simulink model "CUD_10m"  (R2019a)
settings: Solver=VariableStepAuto  StartTime=1.0  StopTime=144  RelTol=1e-3
values from neighbouring files (symbols this model uses):
  altezza = [0,0,0,0,0,0,0,0,0,0,0,0,0,0,0,0,0,0,0,0,0,0,0,0,0,0,0,0,0,0,0,0,0,0,0,0,0,0,0.81,2.62,4.43,6.26,8.1,9.94,11.79,13.65,15.51,17.37,19.23,21.1,22.95,24.81,26.66,28.49,30.32,32.14,33.94,35.73,37.49,39.23,40.94,42.62,44.27,45.87,47.43,48.94,50.39,51.77,53.08,54.3,55.44,56.47,57.39,58.18,58.85,59.37,59.74,59.96,60.02,59.93,59.67,59.27,58.71,58.02,57.2,56.25,55.2,54.05,52.8,51.48,50.08,48.62,47.1,45.53, ...(+192 chars)    [controllo_utenze_domestiche.m]
  area = pi*l_pale^2/4    (= 78.5398163397)    [controllo_utenze_domestiche.m]
  asciugacapelli = utenze(7,:)    [controllo_utenze_domestiche.m]
  azimut = [0,0,0,0,0,0,0,0,0,0,0,0,0,0,0,0,0,0,0,0,0,0,0,0,0,0,0,0,0,0,0,0,0,0,0,0,0,0,74.76,76.41,78.06,79.69,81.32,82.95,84.58,86.21,87.86,89.51,91.18,92.88,94.59,96.34,98.12,99.94,101.81,103.73,105.7,107.74,109.85,112.05,114.33,116.72,119.21,121.83,124.58,127.47,130.51,133.73,137.12,140.7,144.46,148.43,152.58,156.92,161.43,166.09,170.86,175.71,180.61,185.49,190.33,195.08,199.71,204.18,208.48,212.59,216.5 ...(+274 chars)    [controllo_utenze_domestiche.m]
  computer = utenze(9,:)    [controllo_utenze_domestiche.m]
  condizionatori = utenze(4,:)    [controllo_utenze_domestiche.m]
  console = utenze(13,:)    [controllo_utenze_domestiche.m]
  Cp = 0.22    [controllo_utenze_domestiche.m]
  densita = 1.225    [controllo_utenze_domestiche.m]
  fornitura = 3000    [controllo_utenze_domestiche.m]
  forno = utenze(2,:)    [controllo_utenze_domestiche.m]
  frigorifero = utenze(3,:)    [controllo_utenze_domestiche.m]
  irraggiamento = [0,0,0,0,0,0,0,0,0,0,0,0,0,0,0,0,0,0,0,0,0,0,0,0,0,0,0,0,0,0,0,0,0,0,0,0,0,0,0,0,0,0,0,1000,1000,1000,1000,1000,1000,1000,1000,1000,1000,1000,1000,1000,1000,1000,1000,1000,1000,1000,1000,1000,1000,1000,1000,1000,1000,1000,1000,1000,1000,1000,1000,1000,1000,1000,1000,1000,1000,1000,1000,1000,1000,1000,1000,1000,1000,1000,1000,1000,1000,1000,1000,1000,1000,1000,1000,1000,1000,1000,1000,1000,1000,100 ...(+102 chars)    [controllo_utenze_domestiche.m]
  lavastoviglie = utenze(6,:)    [controllo_utenze_domestiche.m]
  lavatrice = utenze(1,:)    [controllo_utenze_domestiche.m]
  luci = utenze(12,:)    [controllo_utenze_domestiche.m]
  microonde = utenze(10,:)    [controllo_utenze_domestiche.m]
  N_cell = 5    [controllo_utenze_domestiche.m]
  N_comp = 3    [controllo_utenze_domestiche.m]
  N_luci = 8    [controllo_utenze_domestiche.m]
  N_pale = 4    [controllo_utenze_domestiche.m]
  N_pann = 10    [controllo_utenze_domestiche.m]
  N_tel = 3    [controllo_utenze_domestiche.m]
  pot_asciu = 2000    [controllo_utenze_domestiche.m]
  pot_comp = 150    [controllo_utenze_domestiche.m]
  pot_cond = 50    [controllo_utenze_domestiche.m]
  pot_cons = 250    [controllo_utenze_domestiche.m]
  pot_forno = 1500    [controllo_utenze_domestiche.m]
  pot_frigo = 25    [controllo_utenze_domestiche.m]
  pot_lav = 2100    [controllo_utenze_domestiche.m]
  pot_lavast = 670    [controllo_utenze_domestiche.m]
  pot_luci = 5    [controllo_utenze_domestiche.m]
  pot_micro = 800    [controllo_utenze_domestiche.m]
  pot_ric = 3    [controllo_utenze_domestiche.m]
  pot_scald = 1500    [controllo_utenze_domestiche.m]
  pot_ste = 150    [controllo_utenze_domestiche.m]
  pot_tel = 55    [controllo_utenze_domestiche.m]
  rend_sol = 0.2    [controllo_utenze_domestiche.m]
  ricariche_cell = utenze(14,:)    [controllo_utenze_domestiche.m]
  scaldabagno = utenze(11,:)    [controllo_utenze_domestiche.m]
  sfasamento = -180    [controllo_utenze_domestiche.m]
  stereo_dvd = utenze(8,:)    [controllo_utenze_domestiche.m]
  sup_pann = 1.5    [controllo_utenze_domestiche.m]
  televisore = utenze(5,:)    [controllo_utenze_domestiche.m]
  vel_vento = [1.3, 1.4, 1.5, 1.7, 1.2, 2.0, 2.1, 1.8, 1.7, 1.5, 1.9, 2.0, 2.2, 2.1, 1.9, 1.7, 1.9, 2.1, 2.2, 2.0, 2.3, 2.1, 2.0, 1.9, 2.1, 2.4, 2.2, 2.2, 2.1, 1.9, 1.5, 1.3, 1.1, 0.9, 1.0, 0.7, 0.8, 0.9, 0.6, 0.9, 1.0, 1.1, 1.2, 1.3, 1.4, 1.2, 1.2, 1.0, 1.2, 1.3, 1.1, 1.5, 1.6, 1.5, 1.4, 1.6, 1.5, 1.3, 1.3, 1.4, 1.2, 1.3, 1.5, 1.6, 1.8, 1.7, 1.7, 1.6, 1.5, 1.6, 1.8, 1.6, 1.5, 1.5, 1.4, 1.3, 1.5, 1.8, 2.1, 2.6, ...(+320 chars)    [controllo_utenze_domestiche.m]
settings Model: Creator=Fernando  LastModifiedBy=Veronica
settings DataIOCC: SaveFormat=StructureWithTime

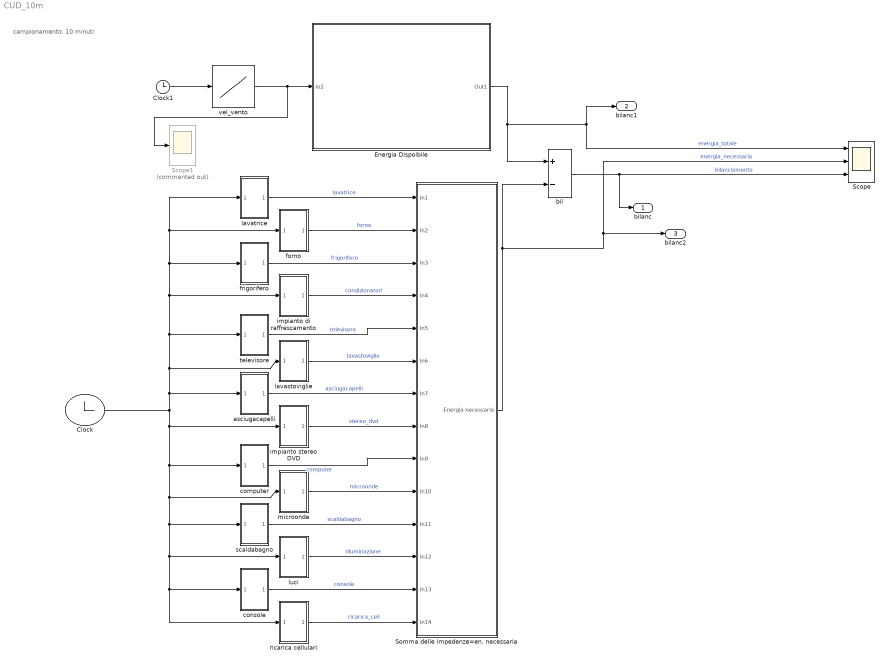
== system CUD_10m ==
  note: campionamento:
      | 10 minuti
  Clock : Clock
  Clock1 : Clock
  Energia Dispoibile : Subsystem
  Scope : Scope  NumInputPorts=3
  Scope1 : Scope  Commented=on
  Somma delle impedenze=en. necessaria : Subsystem  AncestorBlock=modello_progetto_corretto/Somma delle impedenze=en. necessaria
  asciugacapelli : Subsystem
  bil : Sum  Inputs=+-
  computer : Subsystem
  console : Subsystem
  forno : Subsystem
  frigorifero : Subsystem
  impianto di raffrescamento : Subsystem
  impianto stereo DVD : Subsystem
  lavastoviglie : Subsystem
  lavatrice : Subsystem
  luci : Subsystem
  microonde : Subsystem
  ricarica cellulari : Subsystem
  scaldabagno : Subsystem
  televisore : Subsystem
  vel_vento : Lookup_n-D  NumberOfTableDimensions=1  BreakpointsForDimension1=[1:144]  Table=vel_vento  InternalRulePriority=Speed  RndMeth=Simplest  InputSameDT=on
  bilanc : Outport  SampleTime=1
  bilanc1 : Outport  Port=2  SampleTime=1
  bilanc2 : Outport  Port=3  SampleTime=1
  wires:
  vel_vento/1 -> Scope1/1, Energia Dispoibile/1(In2)
  Energia Dispoibile/1(Out1) -> bilanc1/1, Scope/1, bil/1  "energia_totale"
  Somma delle impedenze=en. necessaria/1(Energia necessaria) -> Scope/2, bilanc2/1, bil/2  "energia_necessaria"
  lavatrice/1(Out1) -> Somma delle impedenze=en. necessaria/1(In1)  "lavatrice"
  forno/1(Out1) -> Somma delle impedenze=en. necessaria/2(In2)  "forno"
  frigorifero/1(Out1) -> Somma delle impedenze=en. necessaria/3(In3)  "frigorifero"
  impianto di raffrescamento/1(Out1) -> Somma delle impedenze=en. necessaria/4(In4)  "condizionatori"
  televisore/1(Out1) -> Somma delle impedenze=en. necessaria/5(In5)  "televisore"
  lavastoviglie/1(Out1) -> Somma delle impedenze=en. necessaria/6(In6)  "lavastoviglie"
  asciugacapelli/1(Out1) -> Somma delle impedenze=en. necessaria/7(In7)  "asciugacapelli"
  impianto stereo DVD/1(Out1) -> Somma delle impedenze=en. necessaria/8(In8)  "stereo_dvd"
  computer/1(Out1) -> Somma delle impedenze=en. necessaria/9(In9)  "computer"
  microonde/1(Out1) -> Somma delle impedenze=en. necessaria/10(In10)  "microonde"
  luci/1(Out1) -> Somma delle impedenze=en. necessaria/12(In12)  "illuminazione"
  console/1(Out1) -> Somma delle impedenze=en. necessaria/13(In13)  "console"
  ricarica cellulari/1(Out1) -> Somma delle impedenze=en. necessaria/14(In14)  "ricarica_cell"
  Clock/1 -> televisore/1(In1), frigorifero/1(In1), forno/1(In1), lavatrice/1(In1), impianto di raffrescamento/1(In1), lavastoviglie/1(In1), asciugacapelli/1(In1), impianto stereo DVD/1(In1), computer/1(In1), microonde/1(In1), scaldabagno/1(In1), luci/1(In1), console/1(In1), ricarica cellulari/1(In1)
  bil/1 -> bilanc/1, Scope/3  "bilanciamento"
  Clock1/1 -> vel_vento/1
  scaldabagno/1(Out1) -> Somma delle impedenze=en. necessaria/11(In11)  "scaldabagno"

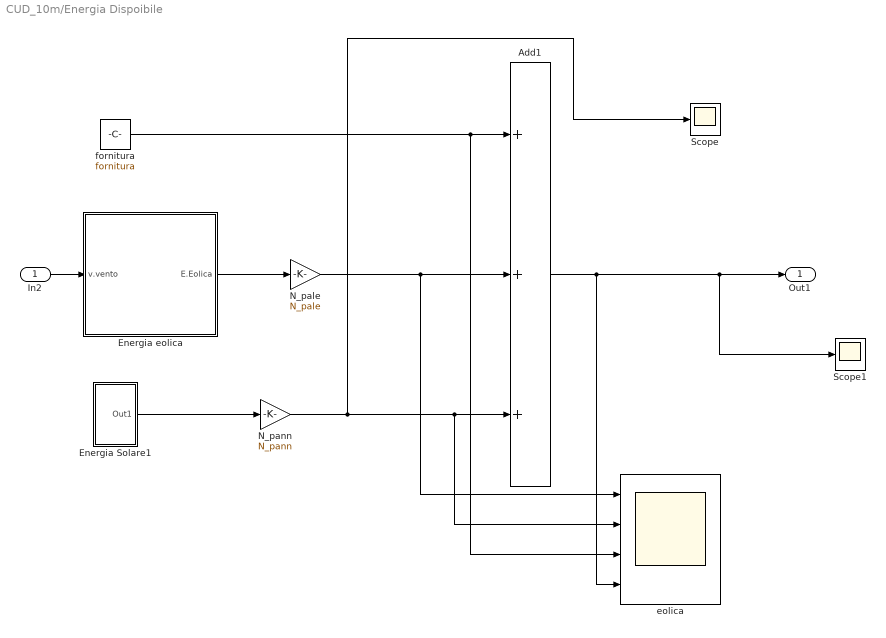
== system CUD_10m/Energia Dispoibile ==
  In2 : Inport
  Add1 : Sum  Inputs=+++
  Energia Solare1 : Subsystem  AncestorBlock=modello_progetto_corretto/calcolo energia ricavata/Energia Solare
  Energia eolica : Subsystem
  N_pale : Gain  Gain=N_pale
  N_pann : Gain  Gain=N_pann
  Scope : Scope
  Scope1 : Scope
  eolica : Scope  NumInputPorts=4
  fornitura : Constant  Value=fornitura
  Out1 : Outport
  wires:
  fornitura/1 -> eolica/3, Add1/1
  Add1/1 -> Scope1/1, Out1/1, eolica/4
  Energia Solare1/1(Out1) -> N_pann/1
  N_pann/1 -> Scope/1, eolica/2, Add1/3
  N_pale/1 -> eolica/1, Add1/2
  In2/1 -> Energia eolica/1(v.vento)
  Energia eolica/1(E.Eolica) -> N_pale/1

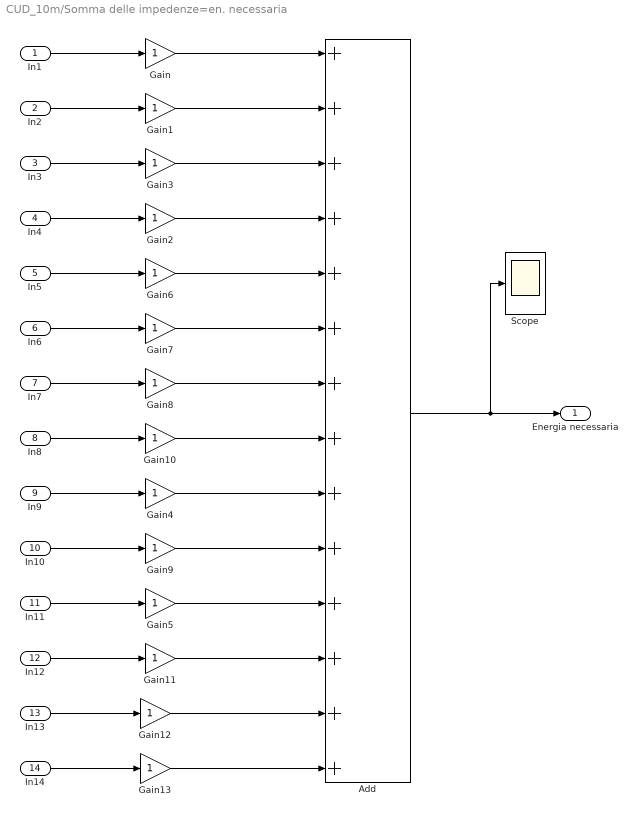
== system CUD_10m/Somma delle impedenze=en. necessaria ==
  In1 : Inport
  In2 : Inport  Port=2
  In3 : Inport  Port=3
  In4 : Inport  Port=4
  In5 : Inport  Port=5
  In6 : Inport  Port=6
  In7 : Inport  Port=7
  In8 : Inport  Port=8
  In9 : Inport  Port=9
  In10 : Inport  Port=10
  In11 : Inport  Port=11
  In12 : Inport  Port=12
  In13 : Inport  Port=13
  In14 : Inport  Port=14
  Add : Sum  Inputs=++++++++++++++
  Gain{,1..13} (14 alike) : Gain
  Scope : Scope
  Energia necessaria : Outport
  wires:
  In7/1 -> Gain8/1
  In8/1 -> Gain10/1
  In10/1 -> Gain9/1
  Gain3/1 -> Add/3
  Gain9/1 -> Add/10
  In3/1 -> Gain3/1
  In2/1 -> Gain1/1
  In4/1 -> Gain2/1
  In1/1 -> Gain/1
  Gain7/1 -> Add/6
  Gain10/1 -> Add/8
  Gain6/1 -> Add/5
  In9/1 -> Gain4/1
  Gain5/1 -> Add/11
  Gain1/1 -> Add/2
  Gain8/1 -> Add/7
  Add/1 -> Scope/1, Energia necessaria/1
  In5/1 -> Gain6/1
  In11/1 -> Gain5/1
  In6/1 -> Gain7/1
  Gain/1 -> Add/1
  Gain2/1 -> Add/4
  Gain4/1 -> Add/9
  In14/1 -> Gain13/1
  In13/1 -> Gain12/1
  In12/1 -> Gain11/1
  Gain11/1 -> Add/12
  Gain12/1 -> Add/13
  Gain13/1 -> Add/14

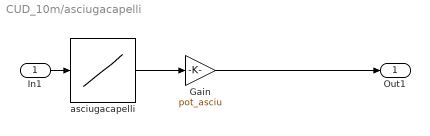
== system CUD_10m/asciugacapelli ==
  In1 : Inport
  Gain : Gain  Gain=pot_asciu
  asciugacapelli : Lookup_n-D  NumberOfTableDimensions=1  BreakpointsForDimension1=[1:144]  Table=asciugacapelli  InternalRulePriority=Speed  RndMeth=Simplest  InputSameDT=on
  Out1 : Outport
  wires:
  asciugacapelli/1 -> Gain/1
  Gain/1 -> Out1/1
  In1/1 -> asciugacapelli/1

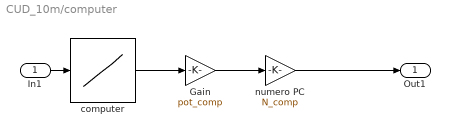
== system CUD_10m/computer ==
  In1 : Inport
  Gain : Gain  Gain=pot_comp
  computer : Lookup_n-D  NumberOfTableDimensions=1  BreakpointsForDimension1=[1:144]  Table=computer  InternalRulePriority=Speed  RndMeth=Simplest  InputSameDT=on
  numero PC : Gain  Gain=N_comp
  Out1 : Outport
  wires:
  computer/1 -> Gain/1
  Gain/1 -> numero PC/1
  In1/1 -> computer/1
  numero PC/1 -> Out1/1

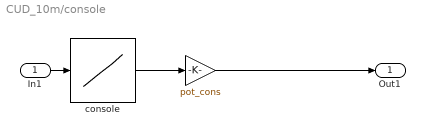
== system CUD_10m/console ==
  In1 : Inport
  " " : Gain  Gain=pot_cons
  console : Lookup_n-D  NumberOfTableDimensions=1  BreakpointsForDimension1=[1:144]  Table=console  InternalRulePriority=Speed  RndMeth=Simplest  InputSameDT=on
  Out1 : Outport
  wires:
  console/1 -> " "/1
  In1/1 -> console/1
  " "/1 -> Out1/1

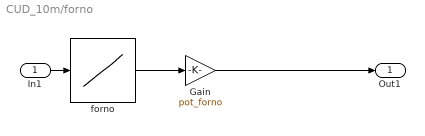
== system CUD_10m/forno ==
  In1 : Inport
  Gain : Gain  Gain=pot_forno
  forno : Lookup_n-D  NumberOfTableDimensions=1  BreakpointsForDimension1=[1:144]  Table=forno  InternalRulePriority=Speed  RndMeth=Simplest  InputSameDT=on
  Out1 : Outport
  wires:
  forno/1 -> Gain/1
  Gain/1 -> Out1/1
  In1/1 -> forno/1

== system CUD_10m/frigorifero ==
  In1 : Inport
  Gain : Gain  Gain=pot_frigo
  frigorifero : Lookup_n-D  NumberOfTableDimensions=1  BreakpointsForDimension1=[1:144]  Table=frigorifero  InternalRulePriority=Speed  RndMeth=Simplest  InputSameDT=on
  Out1 : Outport
  wires:
  frigorifero/1 -> Gain/1
  Gain/1 -> Out1/1
  In1/1 -> frigorifero/1

== system CUD_10m/impianto di raffrescamento ==
  In1 : Inport
  Gain : Gain  Gain=pot_cond
  impianto di raffrescamento : Lookup_n-D  NumberOfTableDimensions=1  BreakpointsForDimension1=[1:144]  Table=condizionatori  InternalRulePriority=Speed  RndMeth=Simplest  InputSameDT=on
  Out1 : Outport
  wires:
  impianto di raffrescamento/1 -> Gain/1
  Gain/1 -> Out1/1
  In1/1 -> impianto di raffrescamento/1

== system CUD_10m/impianto stereo DVD ==
  In1 : Inport
  Gain : Gain  Gain=pot_ste
  impianto stereo DVD : Lookup_n-D  NumberOfTableDimensions=1  BreakpointsForDimension1=[1:144]  Table=stereo_dvd  InternalRulePriority=Speed  RndMeth=Simplest  InputSameDT=on
  Out1 : Outport
  wires:
  impianto stereo DVD/1 -> Gain/1
  Gain/1 -> Out1/1
  In1/1 -> impianto stereo DVD/1

== system CUD_10m/lavastoviglie ==
  In1 : Inport
  Gain : Gain  Gain=pot_lavast
  lavastoviglie : Lookup_n-D  NumberOfTableDimensions=1  BreakpointsForDimension1=[1:144]  Table=lavastoviglie  InternalRulePriority=Speed  RndMeth=Simplest  InputSameDT=on
  Out1 : Outport
  wires:
  lavastoviglie/1 -> Gain/1
  Gain/1 -> Out1/1
  In1/1 -> lavastoviglie/1

== system CUD_10m/lavatrice ==
  In1 : Inport
  Gain : Gain  Gain=pot_lav
  lavatrice : Lookup_n-D  NumberOfTableDimensions=1  BreakpointsForDimension1=[1:144]  Table=lavatrice  InternalRulePriority=Speed  RndMeth=Simplest  InputSameDT=on
  Out1 : Outport
  wires:
  lavatrice/1 -> Gain/1
  Gain/1 -> Out1/1
  In1/1 -> lavatrice/1

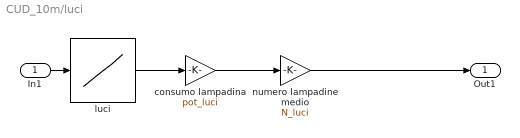
== system CUD_10m/luci ==
  In1 : Inport
  consumo lampadina : Gain  Gain=pot_luci
  luci : Lookup_n-D  NumberOfTableDimensions=1  BreakpointsForDimension1=[1:144]  Table=luci  InternalRulePriority=Speed  RndMeth=Simplest  InputSameDT=on
  numero lampadine medio : Gain  Gain=N_luci
  Out1 : Outport
  wires:
  luci/1 -> consumo lampadina/1
  consumo lampadina/1 -> numero lampadine medio/1
  In1/1 -> luci/1
  numero lampadine medio/1 -> Out1/1

== system CUD_10m/microonde ==
  In1 : Inport
  Gain : Gain  Gain=pot_micro
  microonde : Lookup_n-D  NumberOfTableDimensions=1  BreakpointsForDimension1=[1:144]  Table=microonde  InternalRulePriority=Speed  RndMeth=Simplest  InputSameDT=on
  Out1 : Outport
  wires:
  microonde/1 -> Gain/1
  Gain/1 -> Out1/1
  In1/1 -> microonde/1

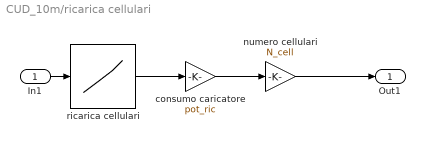
== system CUD_10m/ricarica cellulari ==
  In1 : Inport
  consumo caricatore : Gain  Gain=pot_ric
  numero cellulari : Gain  Gain=N_cell
  ricarica cellulari : Lookup_n-D  NumberOfTableDimensions=1  BreakpointsForDimension1=[1:144]  Table=ricariche_cell  InternalRulePriority=Speed  RndMeth=Simplest  InputSameDT=on
  Out1 : Outport
  wires:
  ricarica cellulari/1 -> consumo caricatore/1
  In1/1 -> ricarica cellulari/1
  consumo caricatore/1 -> numero cellulari/1
  numero cellulari/1 -> Out1/1

== system CUD_10m/scaldabagno ==
  In1 : Inport
  Gain : Gain  Gain=pot_scald
  scaldabagno : Lookup_n-D  NumberOfTableDimensions=1  BreakpointsForDimension1=[1:144]  Table=scaldabagno  InternalRulePriority=Speed  RndMeth=Simplest  InputSameDT=on
  Out1 : Outport
  wires:
  scaldabagno/1 -> Gain/1
  Gain/1 -> Out1/1
  In1/1 -> scaldabagno/1

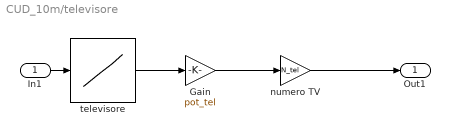
== system CUD_10m/televisore ==
  In1 : Inport
  Gain : Gain  Gain=pot_tel
  numero TV : Gain  Gain=N_tel
  televisore : Lookup_n-D  NumberOfTableDimensions=1  BreakpointsForDimension1=[1:144]  Table=televisore  InternalRulePriority=Speed  RndMeth=Simplest  InputSameDT=on
  Out1 : Outport
  wires:
  televisore/1 -> Gain/1
  Gain/1 -> numero TV/1
  In1/1 -> televisore/1
  numero TV/1 -> Out1/1

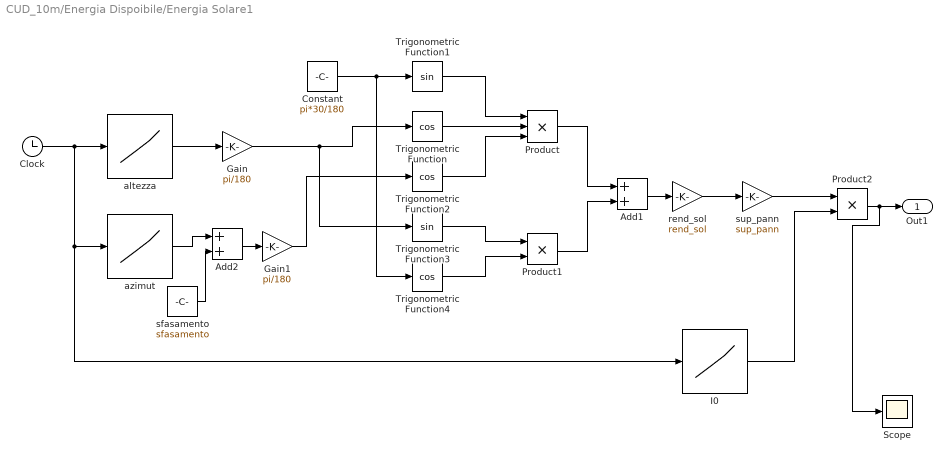
== system CUD_10m/Energia Dispoibile/Energia Solare1 ==
  Add1 : Sum
  Add2 : Sum
  Clock : Clock
  Constant : Constant  Value=pi*30/180
  Gain : Gain  Gain=pi/180
  Gain1 : Gain  Gain=pi/180
  I0 : Lookup_n-D  NumberOfTableDimensions=1  BreakpointsForDimension1=[1:144]  Table=irraggiamento  InternalRulePriority=Speed  RndMeth=Simplest  InputSameDT=on
  Product : Product  Inputs=3
  Product1 : Product
  Product2 : Product
  Scope : Scope
  Trigonometric Function : Trigonometry  Operator=cos
  Trigonometric Function1 : Trigonometry
  Trigonometric Function2 : Trigonometry  Operator=cos
  Trigonometric Function3 : Trigonometry
  Trigonometric Function4 : Trigonometry  Operator=cos
  altezza : Lookup_n-D  NumberOfTableDimensions=1  BreakpointsForDimension1=[1:144]  Table=altezza  InternalRulePriority=Speed  RndMeth=Simplest  InputSameDT=on
  azimut : Lookup_n-D  NumberOfTableDimensions=1  BreakpointsForDimension1=[1:144]  Table=azimut  InternalRulePriority=Speed  RndMeth=Simplest  InputSameDT=on
  rend_sol : Gain  Gain=rend_sol
  sfasamento : Constant  Value=sfasamento
  sup_pann : Gain  Gain=sup_pann
  Out1 : Outport
  wires:
  Trigonometric Function2/1 -> Product/3
  Clock/1 -> I0/1, azimut/1, altezza/1
  Trigonometric Function1/1 -> Product/1
  Gain1/1 -> Trigonometric Function2/1
  rend_sol/1 -> sup_pann/1
  Trigonometric Function4/1 -> Product1/2
  Add2/1 -> Gain1/1
  Constant/1 -> Trigonometric Function4/1, Trigonometric Function1/1
  I0/1 -> Product2/2
  Add1/1 -> rend_sol/1
  Product/1 -> Add1/1
  Product1/1 -> Add1/2
  Trigonometric Function3/1 -> Product1/1
  Gain/1 -> Trigonometric Function3/1, Trigonometric Function/1
  azimut/1 -> Add2/1
  Trigonometric Function/1 -> Product/2
  altezza/1 -> Gain/1
  sfasamento/1 -> Add2/2
  sup_pann/1 -> Product2/1
  Product2/1 -> Scope/1, Out1/1

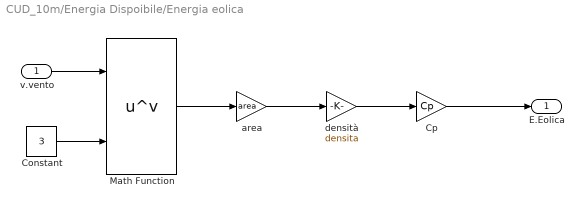
== system CUD_10m/Energia Dispoibile/Energia eolica ==
  v.vento : Inport
  Constant : Constant  Value=3
  Cp : Gain  Gain=Cp
  Math Function : Math  Operator=pow  SaturateOnIntegerOverflow=on
  area : Gain  Gain=area
  densità : Gain  Gain=densita
  E.Eolica : Outport
  wires:
  densità/1 -> Cp/1
  area/1 -> densità/1
  v.vento/1 -> Math Function/1
  Constant/1 -> Math Function/2
  Cp/1 -> E.Eolica/1
  Math Function/1 -> area/1
